simulink model "f2837x_eeprom_emulation"  (R2020b)
settings: Solver=FixedStepDiscrete  StartTime=0.0  StopTime=Inf  FixedStep=1  RelTol=1e-3  EnableMultiTasking=on
undefined symbols (not defined in the file or in its folder): cal_param1_CURRENT_BANK, cal_param2_CURRENT_PAGE, cal_param3_CAL_UPDATE, cal_param4, myParams, xArray
libraries: simulink x3, idelinklib_common x2, demo_controls x1
settings Model: ExtModeTrigDuration=8  Creator=Administrator  LastModifiedBy=User
settings DataIOCC: ReturnWorkspaceOutputs=off
settings OptimizationCC: DefaultUnderspecifiedDataType=single  PassReuseOutputArgsAs=Individual arguments  MaxStackSize=1024  DenormalBehavior=FlushToZero  EfficientTunableParamExpr=on
settings DebuggingCC: InheritedTsInSrcMsg=none  ParameterPrecisionLossMsg=none  ParameterTunabilityLossMsg=error  ArithmeticOperatorsInVariantConditions=warning
settings HardwareCC: ProdBitPerChar=16  ProdBitPerInt=16  ProdBitPerPointer=32  ProdBitPerSizeT=32  ProdBitPerPtrDiffT=32  ProdLargestAtomicInteger=Integer  ProdLargestAtomicFloat=None  ProdWordSize=16  ProdLongLongMode=on  ProdHWDeviceType=Texas Instruments->C2000
settings SFSimCC: SimUseLocalCustomCode=off  MATLABDynamicMemAlloc=off  CustomCodeUndefinedFunction=UseInterfaceOnly
settings RTWCC: Description=Embedded Coder  SystemTargetFile=ert.tlc  HardwareBoard=TI Delfino F28379D LaunchPad  TemplateMakefile=ert_default_tmf  GenerateReport=on  RTWUseLocalCustomCode=off  CustomSource=Fapi_UserDefinedFunctions.c  CustomLibrary=F021_API_F2837xD_FPU32.lib  Toolchain=Texas Instruments Code Composer Studio (C2000)  IncludeHyperlinkInReport=on  LaunchReport=on  GenerateTraceInfo=on  GenerateTraceReport=on  GenerateTraceReportSl=on  GenerateTraceReportSf=on  GenerateTraceReportEml=on
settings RTWCC: CustomHeaderCode=|
  | #include "flash_programming_c28.h"
  | #include "F021_F2837xD_C28x.h"
settings RTWCC: CustomInclude=|
  | C:\ti\controlSUITE\device_support\F2837xD\v190\F2837xD_examples_Dual\flash_programming\cpu01
  | C:\ti\controlSUITE\device_support\F2837xD\v190\F2837xD_common\include\FlashAPI\Constants
  | C:\ti\controlSUITE\device_support\F2837xD\v190\F2837xD_common\include\FlashAPI
  | C:\ti\controlSUITE\device_support\F2837xD\v190\F2837xD_common\lib
settings CodeAppCC: ForceParamTrailComments=on  IgnoreCustomStorageClasses=off  OperatorAnnotations=on  SimulinkDataObjDesc=on  SFDataObjDesc=on  MATLABFcnDesc=on  InsertBlockDesc=on  StateflowObjectComments=on  MATLABSourceComments=on
settings ERTTargetCC: CodeReplacementLibrary=TI C28x  ExtModeTransport=4  ExtModeStaticAllocSize=10000  ExtModeMexFile=ext_xcp  ExtModeIntrfLevel=Level2 - Open  MemSecPackage=Simulink  MemSecDataConstants=MemConst  MemSecDataIO=MemConst  MemSecDataInternal=MemConst  MemSecDataParameters=MemConst

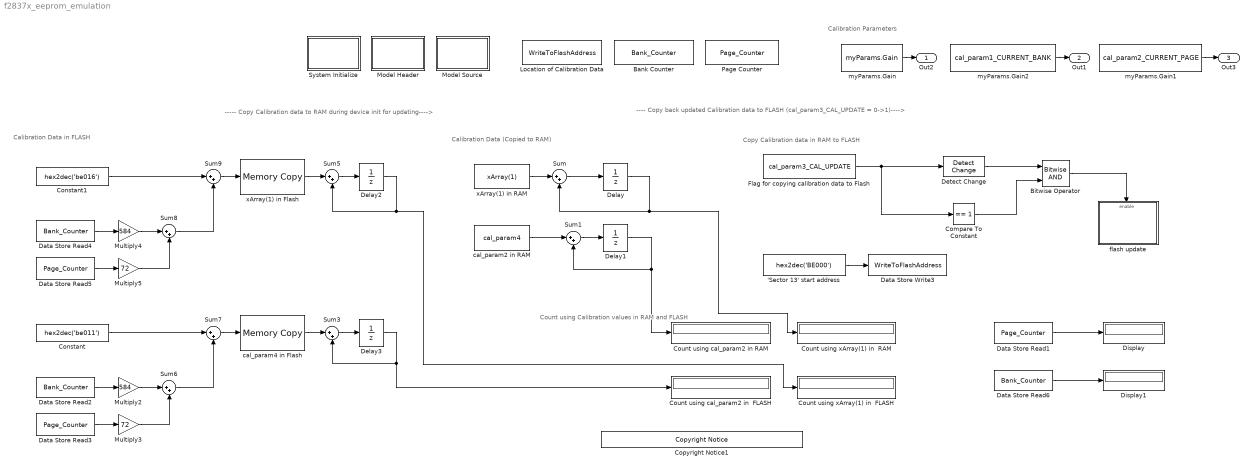
== system f2837x_eeprom_emulation ==
  note: Copy Calibration data in RAM to FLASH
  note: Calibration Data (Copied to RAM)
  note: Calibration Data in FLASH
  note: ----- Copy Calibration data to RAM during device init for updating---->
  note: ---- Copy back updated Calibration data to FLASH (cal_param3_CAL_UPDATE = 0->1)---->
  note: Calibration Parameters
  note: Count using Calibration values in RAM and FLASH
  'Sector 13' start address : Constant  Value=hex2dec('BE000')  OutDataTypeStr=uint32  SampleTime=-1
  Bank Counter : DataStoreMemory  DataStoreName=Bank_Counter  ReadBeforeWriteMsg=warning  WriteAfterWriteMsg=warning  WriteAfterReadMsg=warning  ShowAdditionalParam=off  OutDataTypeStr=uint16  StateMustResolveToSignalObject=on
  Bitwise Operator : simulink/Logic and Bit Operations/Bitwise Operator  logicop=AND  UseBitMask=off  NumInputPorts=2  BitMask=bin2dec('11011001')  BitMaskRealWorld=Stored Integer
  Compare To Constant : simulink/Logic and Bit Operations/Compare To Constant  relop===  const=1  OutDataTypeStr=boolean
  Constant : Constant  Value=hex2dec('be011')  OutDataTypeStr=uint32
  Constant1 : Constant  Value=hex2dec('be016')  OutDataTypeStr=uint32
  Copyright Notice1 : demo_controls/Copyright Notice  year=2021  prod=tic2000
      settings: SourceProductBaseCode=ME
  Count using cal_param2 in  FLASH : Display
  Count using cal_param2 in RAM : Display
  Count using xArray(1) in  FLASH : Display
  Count using xArray(1) in  RAM : Display
  Data Store Read1 : DataStoreRead  DataStoreName=Page_Counter
  Data Store Read2 : DataStoreRead  DataStoreName=Bank_Counter
  Data Store Read3 : DataStoreRead  DataStoreName=Page_Counter
  Data Store Read4 : DataStoreRead  DataStoreName=Bank_Counter
  Data Store Read5 : DataStoreRead  DataStoreName=Page_Counter
  Data Store Read6 : DataStoreRead  DataStoreName=Bank_Counter
  Data Store Write3 : DataStoreWrite  DataStoreName=WriteToFlashAddress
  Delay : UnitDelay  SampleTime=-1  StateName=Counter1  HasFrameUpgradeWarning=on  StateMustResolveToSignalObject=on
  Delay1 : UnitDelay  SampleTime=-1  StateName=Counter2  HasFrameUpgradeWarning=on  StateMustResolveToSignalObject=on
  Delay2 : UnitDelay  HasFrameUpgradeWarning=on
  Delay3 : UnitDelay  HasFrameUpgradeWarning=on
  Detect Change : simulink/Logic and Bit Operations/Detect Change  vinit=1  OutDataTypeStr=boolean
  Display : Display
  Display1 : Display
  Flag for copying calibration data to Flash : Constant  Value=cal_param3_CAL_UPDATE  SampleTime=-1
  Location of Calibration Data : DataStoreMemory  DataStoreName=WriteToFlashAddress  ReadBeforeWriteMsg=warning  WriteAfterWriteMsg=warning  WriteAfterReadMsg=warning  ShowAdditionalParam=off  OutDataTypeStr=uint32  StateMustResolveToSignalObject=on
  Model Header : Subsystem  mask(Model Header){ShowInLibBrowser=0}
      mask prompts: ShowInLibBrowser "Simulink:masks:CustCodeMaskParam1_MP"
      settings: CopyFcn=cccopyfcn(gcb)  OpenFcn=ccopenfcn('Model Header')
      mask Help: eval('feval(''rtwprivate'',''rtwhelpview'',''rtw_model_header_block'')');
      mask Display: disp('Model\nHeader');
  Model Source : Subsystem  mask(Model Source){ShowInLibBrowser=0}
      mask prompts: ShowInLibBrowser "Simulink:masks:CustCodeMaskParam1_MP"
      settings: CopyFcn=cccopyfcn(gcb)  OpenFcn=ccopenfcn('Model Source')
      mask Help: eval('feval(''rtwprivate'',''rtwhelpview'',''rtw_model_source_block'')');
      mask Display: disp('Model\nSource');
  Multiply2 : Gain  Gain=584  OutDataTypeStr=uint16
  Multiply3 : Gain  Gain=72  OutDataTypeStr=uint16
  Multiply4 : Gain  Gain=584  OutDataTypeStr=uint16
  Multiply5 : Gain  Gain=72  OutDataTypeStr=uint16
  Page Counter : DataStoreMemory  DataStoreName=Page_Counter  ReadBeforeWriteMsg=warning  WriteAfterWriteMsg=warning  WriteAfterReadMsg=warning  ShowAdditionalParam=off  OutDataTypeStr=uint16  StateMustResolveToSignalObject=on
  Sum{,1,3,5,7,9} (6 alike) : Sum  Inputs=|++  InputSameDT=on  SaturateOnIntegerOverflow=on  OutDataTypeStr=Inherit: Same as first input
  Sum6 : Sum  Inputs=|++  InputSameDT=on  OutDataTypeStr=uint32  SaturateOnIntegerOverflow=on
  Sum8 : Sum  Inputs=|++  InputSameDT=on  OutDataTypeStr=uint32  SaturateOnIntegerOverflow=on
  System Initialize : Subsystem  mask(System Initialize){ShowInLibBrowser=0}
      mask prompts: ShowInLibBrowser "Simulink:masks:CustCodeMaskParam1_MP"
      settings: CopyFcn=cccopyfcn(gcb)  OpenFcn=ccopenfcn('System Initialize Function')
      mask Help: eval('feval(''rtwprivate'',''rtwhelpview'',''rtw_sys_initialize_block'')');
      mask Display: disp('System\nInitialize');
  cal_param2 in RAM : Constant  Value=cal_param4  SampleTime=-1
  cal_param4 in Flash : idelinklib_common/Memory Copy  copyFrom=Specified address  copyFromAddressSource=Input port  copyFromAddress=hex2dec('000be011')  copyFromSrcCode=myVariableSrc  dataTypeFrom=int16  dataDimensionFrom=1  useOffsetFrom=off  offsetFromSrc=Specify via dialog  offsetFrom=0  strideFrom=1  copyTo=Output port  copyToAddressSource=Specify via dialog  copyToAddress=hex2dec('00002000')  copyToSrcCode=myVariableDst  dataTypeTo=int16  useOffsetTo=off  offsetToSrc=Specify via dialog  offsetTo=0  strideTo=1  sampleTime=-1  useInitValue=off  initValueSrc=Specify constant value  initValue=1  initValueSrcCode=myInitValueVariable  useAsMask=off  maskOperator=bitwise AND  useTermValue=off  termValue=1  isRealtimeEnabled=off  emitCCBeforeWrite=off  CCBeforeWrite=/* Custom Code Before Write*/  emitCCAfterWrite=off  CCAfterWrite=/* Custom Code After Write*/  useDMACopy=off  enableBlockingMode=off
      settings: SourceProductBaseCode=ME
  flash update : Subsystem
  myParams.Gain : Constant  Value=myParams.Gain  VectorParams1D=off  SampleTime=-1
  myParams.Gain1 : Constant  Value=cal_param2_CURRENT_PAGE  VectorParams1D=off  SampleTime=-1
  myParams.Gain2 : Constant  Value=cal_param1_CURRENT_BANK  VectorParams1D=off  SampleTime=-1
  xArray(1) in Flash : idelinklib_common/Memory Copy  copyFrom=Specified address  copyFromAddressSource=Input port  copyFromAddress=hex2dec('000be011')  copyFromSrcCode=myVariableSrc  dataTypeFrom=int16  dataDimensionFrom=1  useOffsetFrom=off  offsetFromSrc=Specify via dialog  offsetFrom=0  strideFrom=1  copyTo=Output port  copyToAddressSource=Specify via dialog  copyToAddress=hex2dec('00002000')  copyToSrcCode=myVariableDst  dataTypeTo=int16  useOffsetTo=off  offsetToSrc=Specify via dialog  offsetTo=0  strideTo=1  sampleTime=-1  useInitValue=off  initValueSrc=Specify constant value  initValue=1  initValueSrcCode=myInitValueVariable  useAsMask=off  maskOperator=bitwise AND  useTermValue=off  termValue=1  isRealtimeEnabled=off  emitCCBeforeWrite=off  CCBeforeWrite=/* Custom Code Before Write*/  emitCCAfterWrite=off  CCAfterWrite=/* Custom Code After Write*/  useDMACopy=off  enableBlockingMode=off
      settings: SourceProductBaseCode=ME
  xArray(1) in RAM : Constant  Value=xArray(1)  SampleTime=-1
  Out2 : Outport
  Out1 : Outport  Port=2
  Out3 : Outport  Port=3
  wires:
  Flag for copying calibration data to Flash/1 -> Detect Change/1, Compare To Constant/1
  Detect Change/1 -> Bitwise Operator/1
  Bitwise Operator/1 -> flash update/Enable
  Compare To Constant/1 -> Bitwise Operator/2
  Delay/1 -> Count using xArray(1) in  RAM/1, Sum/2
  Sum/1 -> Delay/1
  cal_param2 in RAM/1 -> Sum1/1
  Sum1/1 -> Delay1/1
  xArray(1) in RAM/1 -> Sum/1
  Delay1/1 -> Sum1/2, Count using cal_param2 in RAM/1
  Sum3/1 -> Delay3/1
  Delay2/1 -> Sum5/2, Count using xArray(1) in  FLASH/1
  Delay3/1 -> Count using cal_param2 in  FLASH/1, Sum3/2
  'Sector 13' start address/1 -> Data Store Write3/1
  myParams.Gain/1 -> Out2/1
  myParams.Gain2/1 -> Out1/1
  myParams.Gain1/1 -> Out3/1
  Sum5/1 -> Delay2/1
  Data Store Read2/1 -> Multiply2/1
  Multiply2/1 -> Sum6/1
  Multiply3/1 -> Sum6/2
  Data Store Read3/1 -> Multiply3/1
  Sum6/1 -> Sum7/2
  Constant/1 -> Sum7/1
  Sum7/1 -> cal_param4 in Flash/1
  cal_param4 in Flash/1 -> Sum3/1
  Data Store Read4/1 -> Multiply4/1
  Sum8/1 -> Sum9/2
  Constant1/1 -> Sum9/1
  Multiply4/1 -> Sum8/1
  xArray(1) in Flash/1 -> Sum5/1
  Multiply5/1 -> Sum8/2
  Sum9/1 -> xArray(1) in Flash/1
  Data Store Read5/1 -> Multiply5/1
  Data Store Read1/1 -> Display/1
  Data Store Read6/1 -> Display1/1

== system f2837x_eeprom_emulation/Model Header ==

== system f2837x_eeprom_emulation/Model Source ==

== system f2837x_eeprom_emulation/System Initialize ==

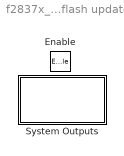
== system f2837x_eeprom_emulation/flash update ==
  Enable : EnablePort
  System Outputs : Subsystem  mask(System Outputs){ShowInLibBrowser=0}
      mask prompts: ShowInLibBrowser "Simulink:masks:CustCodeMaskParam1_MP"
      settings: CopyFcn=cccopyfcn(gcb)  OpenFcn=ccopenfcn('System Outputs Function')
      mask Help: eval('feval(''rtwprivate'',''rtwhelpview'',''rtw_sys_outputs_block'')');
      mask Display: disp('System\nOutputs');

== system f2837x_eeprom_emulation/flash update/System Outputs ==
